simulink model "Task4"  (R2022a)
settings: Solver=FixedStepAuto  StartTime=0.0  StopTime=10.0  FixedStep=0.001  RelTol=1e-3
undefined symbols (not defined in the file): k
settings Model: Creator=Family  LastModifiedBy=Family

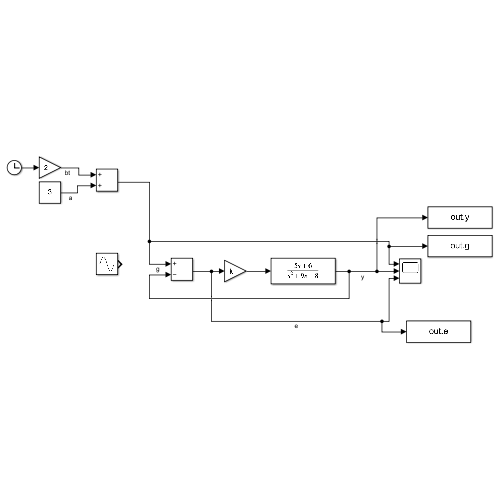
[thumbnail: Simulink's stored preview of the top-level diagram]
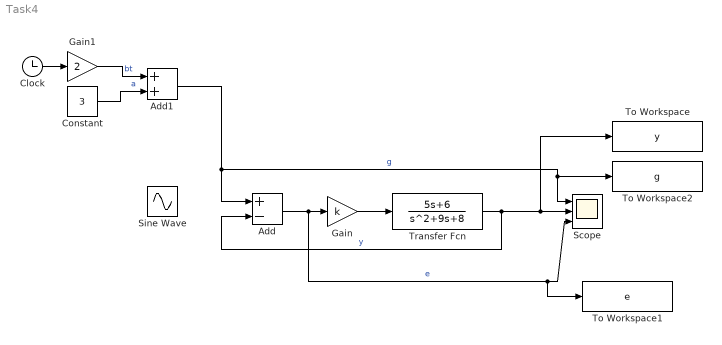
== system Task4 ==
  Add : Sum  Inputs=+-
  Add1 : Sum
  Clock : Clock
  Constant : Constant  Value=3
  Gain : Gain  Gain=k
  Gain1 : Gain  Gain=2
  Scope : Scope  NumInputPorts=3
  Sine Wave : Sin  Amplitude=2  Phase=2  SampleTime=0
  To Workspace : ToWorkspace  VariableName=y  SaveFormat=Timeseries  SampleTime=-1
  To Workspace1 : ToWorkspace  VariableName=e  SaveFormat=Timeseries  SampleTime=-1
  To Workspace2 : ToWorkspace  VariableName=g  SaveFormat=Timeseries  SampleTime=-1
  Transfer Fcn : TransferFcn  Numerator=[5 6]  Denominator=[1 9 8]
  wires:
  Transfer Fcn/1 -> Add/2, To Workspace/1, Scope/2  "y"
  Add/1 -> To Workspace1/1, Scope/3, Gain/1  "e"
  Add1/1 -> Add/1, To Workspace2/1, Scope/1  "g"
  Gain/1 -> Transfer Fcn/1
  Clock/1 -> Gain1/1
  Gain1/1 -> Add1/1  "bt"
  Constant/1 -> Add1/2  "a"
